simulink model "sus"  (Simulink 6.5)
settings: Solver=ode45  StartTime=0.0  StopTime=16  RelTol=1e-3
libraries: cdsFilt x266, cdsBitwise x92, cdsEpicsOut x84, cdsEpicsBinIn x56, cdsEpicsIn x20, cdsFiltCtrl x18, cdsMatrix x11, cdsSwitch x7, cdsWD x7, cdsFunctionCall x5, cdsRio1 x4, dac x3
(part 15 of 20)

== system sus/RLS/DELTA1 ==
  In1 : Inport
  time : Inport  Port=2
  delay_in : Inport  Port=3
  HOLD : Subsystem
  Sum2 : Sum  Inputs=+-
  dy1 : Outport
  delay_out : Outport  Port=2
  wires:
  HOLD/1(out) -> Sum2/2
  In1/1 -> Sum2/1, HOLD/1(In1)
  Sum2/1 -> dy1/1
  time/1 -> HOLD/2(time)
  HOLD/2(delay_out) -> delay_out/1
  delay_in/1 -> HOLD/3(delay_in)

== system sus/RLS/DELTA2 ==
  In1 : Inport
  time : Inport  Port=2
  delay_in : Inport  Port=3
  HOLD : Subsystem
  Sum2 : Sum  Inputs=+-
  dy1 : Outport
  delay_out : Outport  Port=2
  wires:
  HOLD/1(out) -> Sum2/2
  In1/1 -> Sum2/1, HOLD/1(In1)
  Sum2/1 -> dy1/1
  time/1 -> HOLD/2(time)
  HOLD/2(delay_out) -> delay_out/1
  delay_in/1 -> HOLD/3(delay_in)

== system sus/RLS/DELTA3 ==
  In1 : Inport
  time : Inport  Port=2
  delay_in : Inport  Port=3
  HOLD : Subsystem
  Sum2 : Sum  Inputs=+-
  dy1 : Outport
  delay_out : Outport  Port=2
  wires:
  HOLD/1(out) -> Sum2/2
  In1/1 -> Sum2/1, HOLD/1(In1)
  Sum2/1 -> dy1/1
  time/1 -> HOLD/2(time)
  HOLD/2(delay_out) -> delay_out/1
  delay_in/1 -> HOLD/3(delay_in)

== system sus/RLS/J11 ==
  In1 : Inport
  time : Inport  Port=2
  sattime : Inport  Port=3
  delay_in : Inport  Port=4
  Choice2 : Switch  Threshold=0.5
  HOLD : Subsystem
  SR : Constant  Value=0
  Sum2 : Sum
  out : Outport
  delay_out : Outport  Port=2
  wires:
  time/1 -> HOLD/2(time)
  HOLD/2(delay_out) -> delay_out/1
  delay_in/1 -> HOLD/3(delay_in)
  In1/1 -> Sum2/1
  Sum2/1 -> HOLD/1(In1)
  HOLD/1(out) -> Choice2/1
  sattime/1 -> Choice2/2
  Choice2/1 -> out/1, Sum2/2
  SR/1 -> Choice2/3

== system sus/RLS/J12 ==
  In1 : Inport
  time : Inport  Port=2
  sattime : Inport  Port=3
  delay_in : Inport  Port=4
  Choice2 : Switch  Threshold=0.5
  HOLD : Subsystem
  SR : Constant  Value=0
  Sum2 : Sum
  out : Outport
  delay_out : Outport  Port=2
  wires:
  time/1 -> HOLD/2(time)
  HOLD/2(delay_out) -> delay_out/1
  delay_in/1 -> HOLD/3(delay_in)
  In1/1 -> Sum2/1
  Sum2/1 -> HOLD/1(In1)
  HOLD/1(out) -> Choice2/1
  sattime/1 -> Choice2/2
  Choice2/1 -> out/1, Sum2/2
  SR/1 -> Choice2/3

== system sus/RLS/J21 ==
  In1 : Inport
  time : Inport  Port=2
  sattime : Inport  Port=3
  delay_in : Inport  Port=4
  Choice2 : Switch  Threshold=0.5
  HOLD : Subsystem
  SR : Constant  Value=0
  Sum2 : Sum
  out : Outport
  delay_out : Outport  Port=2
  wires:
  time/1 -> HOLD/2(time)
  HOLD/2(delay_out) -> delay_out/1
  delay_in/1 -> HOLD/3(delay_in)
  In1/1 -> Sum2/1
  Sum2/1 -> HOLD/1(In1)
  HOLD/1(out) -> Choice2/1
  sattime/1 -> Choice2/2
  Choice2/1 -> out/1, Sum2/2
  SR/1 -> Choice2/3

== system sus/RLS/J22 ==
  In1 : Inport
  time : Inport  Port=2
  sattime : Inport  Port=3
  delay_in : Inport  Port=4
  Choice2 : Switch  Threshold=0.5
  HOLD : Subsystem
  SR : Constant  Value=0
  Sum2 : Sum
  out : Outport
  delay_out : Outport  Port=2
  wires:
  time/1 -> HOLD/2(time)
  HOLD/2(delay_out) -> delay_out/1
  delay_in/1 -> HOLD/3(delay_in)
  In1/1 -> Sum2/1
  Sum2/1 -> HOLD/1(In1)
  HOLD/1(out) -> Choice2/1
  sattime/1 -> Choice2/2
  Choice2/1 -> out/1, Sum2/2
  SR/1 -> Choice2/3

== system sus/RLS/J31 ==
  In1 : Inport
  time : Inport  Port=2
  sattime : Inport  Port=3
  delay_in : Inport  Port=4
  Choice2 : Switch  Threshold=0.5
  HOLD : Subsystem
  SR : Constant  Value=0
  Sum2 : Sum
  out : Outport
  delay_out : Outport  Port=2
  wires:
  time/1 -> HOLD/2(time)
  HOLD/2(delay_out) -> delay_out/1
  delay_in/1 -> HOLD/3(delay_in)
  In1/1 -> Sum2/1
  Sum2/1 -> HOLD/1(In1)
  HOLD/1(out) -> Choice2/1
  sattime/1 -> Choice2/2
  Choice2/1 -> out/1, Sum2/2
  SR/1 -> Choice2/3

== system sus/RLS/J32 ==
  In1 : Inport
  time : Inport  Port=2
  sattime : Inport  Port=3
  delay_in : Inport  Port=4
  Choice2 : Switch  Threshold=0.5
  HOLD : Subsystem
  SR : Constant  Value=0
  Sum2 : Sum
  out : Outport
  delay_out : Outport  Port=2
  wires:
  time/1 -> HOLD/2(time)
  HOLD/2(delay_out) -> delay_out/1
  delay_in/1 -> HOLD/3(delay_in)
  In1/1 -> Sum2/1
  Sum2/1 -> HOLD/1(In1)
  HOLD/1(out) -> Choice2/1
  sattime/1 -> Choice2/2
  Choice2/1 -> out/1, Sum2/2
  SR/1 -> Choice2/3

== system sus/RLS/JHATDTHETA ==
  11 : Inport
  12 : Inport  Port=2
  21 : Inport  Port=3
  22 : Inport  Port=4
  31 : Inport  Port=5
  32 : Inport  Port=6
  dtheta1 : Inport  Port=7
  dtheta2 : Inport  Port=8
  Product{,1..5} (6 alike) : Product  RndMeth=Zero
  Sum : Sum  Inputs=|++
  Sum1 : Sum  Inputs=|++
  Sum2 : Sum  Inputs=|++
  dy1_hat : Outport
  dy2_hat : Outport  Port=2
  dy3_hat : Outport  Port=3
  wires:
  Product/1 -> Sum/1
  Sum/1 -> dy1_hat/1
  Product1/1 -> Sum/2
  Product2/1 -> Sum1/1
  Sum1/1 -> dy2_hat/1
  Product3/1 -> Sum1/2
  Product4/1 -> Sum2/1
  Sum2/1 -> dy3_hat/1
  Product5/1 -> Sum2/2
  dtheta1/1 -> Product/1, Product2/1, Product4/1
  dtheta2/1 -> Product1/1, Product3/1, Product5/1
  11/1 -> Product/2
  12/1 -> Product1/2
  21/1 -> Product2/2
  22/1 -> Product3/2
  31/1 -> Product4/2
  32/1 -> Product5/2

== system sus/RLS/K1 ==
  P11 : Inport
  P12 : Inport  Port=2
  P21 : Inport  Port=3
  P22 : Inport  Port=4
  dtheta1 : Inport  Port=5
  dtheta2 : Inport  Port=6
  lambda : Inport  Port=7
  Divide : Product  Inputs=*/  OutScaling=2^-10
  Divide1 : Product  Inputs=*/  OutScaling=2^-10
  PDTHETA : Subsystem
  Product : Product  RndMeth=Zero
  Product1 : Product  RndMeth=Zero
  Sum : Sum  Inputs=|+++
  K1_1 : Outport
  K1_2 : Outport  Port=2
  wires:
  P11/1 -> PDTHETA/1(P11)
  P12/1 -> PDTHETA/2(P12)
  P21/1 -> PDTHETA/3(P21)
  P22/1 -> PDTHETA/4(P22)
  dtheta1/1 -> PDTHETA/5(dtheta1), Product/2
  dtheta2/1 -> PDTHETA/6(dtheta2), Product1/2
  PDTHETA/1(out1) -> Product/1, Divide/1
  PDTHETA/2(out2) -> Product1/1, Divide1/1
  Product1/1 -> Sum/2
  Product/1 -> Sum/1
  lambda/1 -> Sum/3
  Sum/1 -> Divide/2, Divide1/2
  Divide/1 -> K1_1/1
  Divide1/1 -> K1_2/1

== system sus/RLS/K2 ==
  P11 : Inport
  P12 : Inport  Port=2
  P21 : Inport  Port=3
  P22 : Inport  Port=4
  dtheta1 : Inport  Port=5
  dtheta2 : Inport  Port=6
  lambda : Inport  Port=7
  Divide : Product  Inputs=*/  OutScaling=2^-10
  Divide1 : Product  Inputs=*/  OutScaling=2^-10
  PDTHETA : Subsystem
  Product : Product  RndMeth=Zero
  Product1 : Product  RndMeth=Zero
  Sum : Sum  Inputs=|+++
  K2_1 : Outport
  K2_2 : Outport  Port=2
  wires:
  P11/1 -> PDTHETA/1(P11)
  P12/1 -> PDTHETA/2(P12)
  P21/1 -> PDTHETA/3(P21)
  P22/1 -> PDTHETA/4(P22)
  dtheta1/1 -> PDTHETA/5(dtheta1), Product/2
  dtheta2/1 -> PDTHETA/6(dtheta2), Product1/2
  PDTHETA/1(out1) -> Product/1, Divide/1
  PDTHETA/2(out2) -> Product1/1, Divide1/1
  Product1/1 -> Sum/2
  Product/1 -> Sum/1
  lambda/1 -> Sum/3
  Sum/1 -> Divide/2, Divide1/2
  Divide/1 -> K2_1/1
  Divide1/1 -> K2_2/1

== system sus/RLS/K3 ==
  P11 : Inport
  P12 : Inport  Port=2
  P21 : Inport  Port=3
  P22 : Inport  Port=4
  dtheta1 : Inport  Port=5
  dtheta2 : Inport  Port=6
  lambda : Inport  Port=7
  Divide : Product  Inputs=*/  OutScaling=2^-10
  Divide1 : Product  Inputs=*/  OutScaling=2^-10
  PDTHETA : Subsystem
  Product : Product  RndMeth=Zero
  Product1 : Product  RndMeth=Zero
  Sum : Sum  Inputs=|+++
  K3_1 : Outport
  K3_2 : Outport  Port=2
  wires:
  P11/1 -> PDTHETA/1(P11)
  P12/1 -> PDTHETA/2(P12)
  P21/1 -> PDTHETA/3(P21)
  P22/1 -> PDTHETA/4(P22)
  dtheta1/1 -> PDTHETA/5(dtheta1), Product/2
  dtheta2/1 -> PDTHETA/6(dtheta2), Product1/2
  PDTHETA/1(out1) -> Product/1, Divide/1
  PDTHETA/2(out2) -> Product1/1, Divide1/1
  Product1/1 -> Sum/2
  Product/1 -> Sum/1
  lambda/1 -> Sum/3
  Sum/1 -> Divide/2, Divide1/2
  Divide/1 -> K3_1/1
  Divide1/1 -> K3_2/1

== system sus/RLS/P1 ==
  note: I - K*dtheta'
  note: (I - K*dtheta')*P
  K1_1 : Inport
  K1_2 : Inport  Port=2
  dtheta1 : Inport  Port=3
  dtheta2 : Inport  Port=4
  time : Inport  Port=5
  sattime : Inport  Port=6
  lambda : Inport  Port=7
  delay_In1 : Inport  Port=8
  delay_In2 : Inport  Port=9
  delay_In3 : Inport  Port=10
  delay_In4 : Inport  Port=11
  Choice{1..4} (4 alike) : Switch  Threshold=0.5
  Divide : Product  Inputs=*/  OutScaling=2^-10
  HOLD : Subsystem
  HOLD1 : Subsystem
  HOLD2 : Subsystem
  HOLD3 : Subsystem
  MATH : Subsystem
  MATH1 : Subsystem
  Product{1..4} (4 alike) : Product  RndMeth=Zero
  SR : Constant  Value=7
  SR1 : Constant  Value=0
  SR2 : Constant  Value=7
  SR3 : Constant  Value=0
  SR4 : Constant
  P1_11 : Outport
  P1_12 : Outport  Port=2
  P1_21 : Outport  Port=3
  P1_22 : Outport  Port=4
  delay_out1 : Outport  Port=5
  delay_out2 : Outport  Port=6
  delay_out3 : Outport  Port=7
  delay_out4 : Outport  Port=8
  wires:
  K1_1/1 -> MATH/1(K1_1)
  K1_2/1 -> MATH/2(K1_2)
  dtheta1/1 -> MATH/3(dtheta1)
  dtheta2/1 -> MATH/4(dtheta2)
  MATH/1(out11) -> MATH1/1(in11)
  MATH/2(out12) -> MATH1/2(in12)
  MATH/3(out21) -> MATH1/3(in21)
  MATH/4(out22) -> MATH1/4(in22)
  Choice2/1 -> HOLD/1(In1)
  sattime/1 -> Choice2/2, Choice1/2, Choice3/2, Choice4/2
  SR/1 -> Choice2/3
  MATH1/1(outP11) -> Choice2/1
  time/1 -> HOLD/2(time), HOLD2/2(time), HOLD3/2(time), HOLD1/2(time)
  Choice1/1 -> HOLD1/1(In1)
  SR1/1 -> Choice1/3
  MATH1/2(outP12) -> Choice1/1
  Choice4/1 -> HOLD2/1(In1)
  SR2/1 -> Choice4/3
  MATH1/3(outP21) -> Choice4/1
  Choice3/1 -> HOLD3/1(In1)
  SR3/1 -> Choice3/3
  MATH1/4(outP22) -> Choice3/1
  SR4/1 -> Divide/1
  lambda/1 -> Divide/2
  HOLD/1(out) -> Product2/2, P1_11/1
  HOLD1/1(out) -> Product1/2, P1_12/1
  HOLD2/1(out) -> Product3/2, P1_21/1
  HOLD3/1(out) -> Product4/2, P1_22/1
  Divide/1 -> Product2/1, Product1/1, Product4/1, Product3/1
  Product2/1 -> MATH1/5(P11)
  Product4/1 -> MATH1/8(P22)
  Product3/1 -> MATH1/7(P21)
  Product1/1 -> MATH1/6(P12)
  delay_In1/1 -> HOLD/3(delay_in)
  delay_In2/1 -> HOLD1/3(delay_in)
  delay_In3/1 -> HOLD2/3(delay_in)
  delay_In4/1 -> HOLD3/3(delay_in)
  HOLD/2(delay_out) -> delay_out1/1
  HOLD1/2(delay_out) -> delay_out2/1
  HOLD2/2(delay_out) -> delay_out3/1
  HOLD3/2(delay_out) -> delay_out4/1

== system sus/RLS/P2 ==
  note: I - K*dtheta'
  note: (I - K*dtheta')*P
  K1_1 : Inport
  K1_2 : Inport  Port=2
  dtheta1 : Inport  Port=3
  dtheta2 : Inport  Port=4
  time : Inport  Port=5
  sattime : Inport  Port=6
  lambda : Inport  Port=7
  delay_In1 : Inport  Port=8
  delay_In2 : Inport  Port=9
  delay_In3 : Inport  Port=10
  delay_In4 : Inport  Port=11
  Choice{1..4} (4 alike) : Switch  Threshold=0.5
  Divide : Product  Inputs=*/  OutScaling=2^-10
  HOLD : Subsystem
  HOLD1 : Subsystem
  HOLD2 : Subsystem
  HOLD3 : Subsystem
  MATH : Subsystem
  MATH1 : Subsystem
  Product{1..4} (4 alike) : Product  RndMeth=Zero
  SR : Constant  Value=7
  SR1 : Constant  Value=0
  SR2 : Constant  Value=7
  SR3 : Constant  Value=0
  SR4 : Constant
  P1_11 : Outport
  P1_12 : Outport  Port=2
  P1_21 : Outport  Port=3
  P1_22 : Outport  Port=4
  delay_out1 : Outport  Port=5
  delay_out2 : Outport  Port=6
  delay_out3 : Outport  Port=7
  delay_out4 : Outport  Port=8
  wires:
  K1_1/1 -> MATH/1(K1_1)
  K1_2/1 -> MATH/2(K1_2)
  dtheta1/1 -> MATH/3(dtheta1)
  dtheta2/1 -> MATH/4(dtheta2)
  MATH/1(out11) -> MATH1/1(in11)
  MATH/2(out12) -> MATH1/2(in12)
  MATH/3(out21) -> MATH1/3(in21)
  MATH/4(out22) -> MATH1/4(in22)
  Choice2/1 -> HOLD/1(In1)
  sattime/1 -> Choice2/2, Choice1/2, Choice3/2, Choice4/2
  SR/1 -> Choice2/3
  MATH1/1(outP11) -> Choice2/1
  time/1 -> HOLD/2(time), HOLD2/2(time), HOLD3/2(time), HOLD1/2(time)
  Choice1/1 -> HOLD1/1(In1)
  SR1/1 -> Choice1/3
  MATH1/2(outP12) -> Choice1/1
  Choice4/1 -> HOLD2/1(In1)
  SR2/1 -> Choice4/3
  MATH1/3(outP21) -> Choice4/1
  Choice3/1 -> HOLD3/1(In1)
  SR3/1 -> Choice3/3
  MATH1/4(outP22) -> Choice3/1
  SR4/1 -> Divide/1
  lambda/1 -> Divide/2
  HOLD/1(out) -> Product2/2, P1_11/1
  HOLD1/1(out) -> Product1/2, P1_12/1
  HOLD2/1(out) -> Product3/2, P1_21/1
  HOLD3/1(out) -> Product4/2, P1_22/1
  Divide/1 -> Product2/1, Product1/1, Product4/1, Product3/1
  Product2/1 -> MATH1/5(P11)
  Product4/1 -> MATH1/8(P22)
  Product3/1 -> MATH1/7(P21)
  Product1/1 -> MATH1/6(P12)
  delay_In1/1 -> HOLD/3(delay_in)
  delay_In2/1 -> HOLD1/3(delay_in)
  delay_In3/1 -> HOLD2/3(delay_in)
  delay_In4/1 -> HOLD3/3(delay_in)
  HOLD/2(delay_out) -> delay_out1/1
  HOLD1/2(delay_out) -> delay_out2/1
  HOLD2/2(delay_out) -> delay_out3/1
  HOLD3/2(delay_out) -> delay_out4/1

== system sus/RLS/P3 ==
  note: I - K*dtheta'
  note: (I - K*dtheta')*P
  K1_1 : Inport
  K1_2 : Inport  Port=2
  dtheta1 : Inport  Port=3
  dtheta2 : Inport  Port=4
  time : Inport  Port=5
  sattime : Inport  Port=6
  lambda : Inport  Port=7
  delay_In1 : Inport  Port=8
  delay_In2 : Inport  Port=9
  delay_In3 : Inport  Port=10
  delay_In4 : Inport  Port=11
  Choice{1..4} (4 alike) : Switch  Threshold=0.5
  Divide : Product  Inputs=*/  OutScaling=2^-10
  HOLD : Subsystem
  HOLD1 : Subsystem
  HOLD2 : Subsystem
  HOLD3 : Subsystem
  MATH : Subsystem
  MATH1 : Subsystem
  Product{1..4} (4 alike) : Product  RndMeth=Zero
  SR : Constant  Value=7
  SR1 : Constant  Value=0
  SR2 : Constant  Value=7
  SR3 : Constant  Value=0
  SR4 : Constant
  P1_11 : Outport
  P1_12 : Outport  Port=2
  P1_21 : Outport  Port=3
  P1_22 : Outport  Port=4
  delay_out1 : Outport  Port=5
  delay_out2 : Outport  Port=6
  delay_out3 : Outport  Port=7
  delay_out4 : Outport  Port=8
  wires:
  K1_1/1 -> MATH/1(K1_1)
  K1_2/1 -> MATH/2(K1_2)
  dtheta1/1 -> MATH/3(dtheta1)
  dtheta2/1 -> MATH/4(dtheta2)
  MATH/1(out11) -> MATH1/1(in11)
  MATH/2(out12) -> MATH1/2(in12)
  MATH/3(out21) -> MATH1/3(in21)
  MATH/4(out22) -> MATH1/4(in22)
  Choice2/1 -> HOLD/1(In1)
  sattime/1 -> Choice2/2, Choice1/2, Choice3/2, Choice4/2
  SR/1 -> Choice2/3
  MATH1/1(outP11) -> Choice2/1
  time/1 -> HOLD/2(time), HOLD2/2(time), HOLD3/2(time), HOLD1/2(time)
  Choice1/1 -> HOLD1/1(In1)
  SR1/1 -> Choice1/3
  MATH1/2(outP12) -> Choice1/1
  Choice4/1 -> HOLD2/1(In1)
  SR2/1 -> Choice4/3
  MATH1/3(outP21) -> Choice4/1
  Choice3/1 -> HOLD3/1(In1)
  SR3/1 -> Choice3/3
  MATH1/4(outP22) -> Choice3/1
  SR4/1 -> Divide/1
  lambda/1 -> Divide/2
  HOLD/1(out) -> Product2/2, P1_11/1
  HOLD1/1(out) -> Product1/2, P1_12/1
  HOLD2/1(out) -> Product3/2, P1_21/1
  HOLD3/1(out) -> Product4/2, P1_22/1
  Divide/1 -> Product2/1, Product1/1, Product4/1, Product3/1
  Product2/1 -> MATH1/5(P11)
  Product4/1 -> MATH1/8(P22)
  Product3/1 -> MATH1/7(P21)
  Product1/1 -> MATH1/6(P12)
  delay_In1/1 -> HOLD/3(delay_in)
  delay_In2/1 -> HOLD1/3(delay_in)
  delay_In3/1 -> HOLD2/3(delay_in)
  delay_In4/1 -> HOLD3/3(delay_in)
  HOLD/2(delay_out) -> delay_out1/1
  HOLD1/2(delay_out) -> delay_out2/1
  HOLD2/2(delay_out) -> delay_out3/1
  HOLD3/2(delay_out) -> delay_out4/1

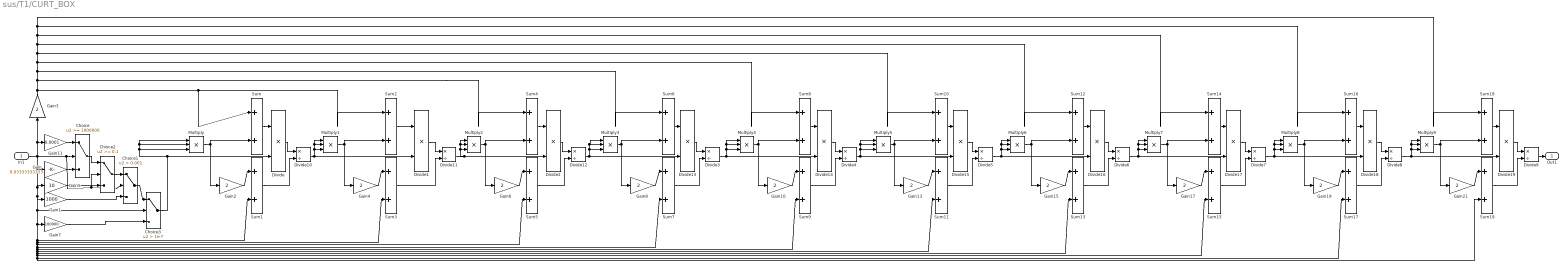
== system sus/T1/CURT_BOX ==
  In1 : Inport
  Choice : Switch  Threshold=1000000
  Choice1 : Switch  Criteria=u2 > Threshold  Threshold=0.001
  Choice2 : Switch  Threshold=0.1
  Choice3 : Switch  Criteria=u2 > Threshold  Threshold=1e-7
  Divide{,1..2,13..19} (10 alike) : Product  Inputs=**  OutScaling=2^-10
  Divide{3..12} (10 alike) : Product  Inputs=*/  OutScaling=2^-10
  Gain : Gain  Gain=0.03333333333
  Gain1 : Gain  Gain=1000
  Gain{2,4,6,8,10,13,15,17,19,21} (10 alike) : Gain  Gain=2
  Gain11 : Gain  Gain=0.0001
  Gain3 : Gain  Orientation=up  Gain=2
  Gain5 : Gain  Gain=10
  Gain7 : Gain  Gain=100000
  Multiply{,1..9} (10 alike) : Product  Inputs=***  OutScaling=2^-10
  Sum{,1..19} (20 alike) : Sum  Inputs=|++
  Out1 : Outport
  wires:
  In1/1 -> Gain/1, Gain1/1, Choice3/2, Sum1/2, Sum3/2, Sum5/2, Sum7/2, Sum9/2, Sum11/2, Sum13/2, Sum15/2, Sum17/2, Sum19/2, Gain7/1, Gain5/1, Choice/2, Choice2/2, Choice1/2, Gain11/1, Gain3/1
  Divide9/1 -> Out1/1
  Gain/1 -> Choice/3
  Gain11/1 -> Choice/1
  Choice3/1 -> Divide/2, Multiply/1, Multiply/2, Multiply/3
  Sum/1 -> Divide/1
  Multiply/1 -> Sum/2, Gain2/1
  Sum1/1 -> Divide10/2
  Gain2/1 -> Sum1/1
  Sum2/1 -> Divide1/1
  Multiply1/1 -> Sum2/2, Gain4/1
  Sum3/1 -> Divide11/2
  Gain4/1 -> Sum3/1
  Sum4/1 -> Divide2/1
  Multiply2/1 -> Sum4/2, Gain6/1
  Gain6/1 -> Sum5/1
  Divide12/1 -> Multiply3/1, Multiply3/2, Multiply3/3, Divide13/2
  Sum6/1 -> Divide13/1
  Multiply3/1 -> Sum6/2, Gain8/1
  Sum7/1 -> Divide3/2
  Gain8/1 -> Sum7/1
  Divide3/1 -> Multiply4/1, Multiply4/2, Multiply4/3, Divide14/2
  Sum8/1 -> Divide14/1
  Multiply4/1 -> Sum8/2, Gain10/1
  Sum9/1 -> Divide4/2
  Gain10/1 -> Sum9/1
  Divide4/1 -> Multiply5/1, Multiply5/2, Multiply5/3, Divide15/2
  Sum10/1 -> Divide15/1
  Multiply5/1 -> Sum10/2, Gain13/1
  Sum11/1 -> Divide5/2
  Gain13/1 -> Sum11/1
  Sum12/1 -> Divide16/1
  Multiply6/1 -> Sum12/2, Gain15/1
  Sum13/1 -> Divide6/2
  Gain15/1 -> Sum13/1
  Sum14/1 -> Divide17/1
  Multiply7/1 -> Sum14/2, Gain17/1
  Sum15/1 -> Divide7/2
  Gain17/1 -> Sum15/1
  Sum16/1 -> Divide18/1
  Multiply8/1 -> Sum16/2, Gain19/1
  Sum17/1 -> Divide8/2
  Gain19/1 -> Sum17/1
  Sum18/1 -> Divide19/1
  Multiply9/1 -> Sum18/2, Gain21/1
  Sum19/1 -> Divide9/2
  Gain21/1 -> Sum19/1
  Gain3/1 -> Sum16/1, Sum18/1, Sum14/1, Sum12/1, Sum10/1, Sum8/1, Sum6/1, Sum4/1, Sum2/1, Sum/1
  Divide/1 -> Divide10/1
  Divide10/1 -> Multiply1/1, Multiply1/2, Multiply1/3, Divide1/2
  Divide11/1 -> Divide2/2, Multiply2/1, Multiply2/2, Multiply2/3
  Divide1/1 -> Divide11/1
  Divide2/1 -> Divide12/1
  Sum5/1 -> Divide12/2
  Divide13/1 -> Divide3/1
  Divide14/1 -> Divide4/1
  Divide15/1 -> Divide5/1
  Divide5/1 -> Multiply6/1, Multiply6/2, Multiply6/3, Divide16/2
  Divide16/1 -> Divide6/1
  Divide6/1 -> Multiply7/1, Multiply7/2, Multiply7/3, Divide17/2
  Divide17/1 -> Divide7/1
  Divide7/1 -> Multiply8/1, Multiply8/2, Multiply8/3, Divide18/2
  Divide18/1 -> Divide8/1
  Divide8/1 -> Multiply9/1, Multiply9/2, Multiply9/3, Divide19/2
  Divide19/1 -> Divide9/1
  Gain1/1 -> Choice1/3
  Choice2/1 -> Choice1/1
  Choice/1 -> Choice2/1
  Gain5/1 -> Choice2/3
  Choice1/1 -> Choice3/1
  Gain7/1 -> Choice3/3

== system sus/T1/E2S ==
  In1 : Inport
  In2 : Inport  Port=2
  In3 : Inport  Port=3
  CONST1 : Constant
  CONST2 : Constant  Value=0
  CONST4 : Constant
  CONST5 : Constant  Value=0
  Choice1 : Switch  Criteria=u2 > Threshold  Threshold=0.0001
  Choice2 : Switch  Criteria=u2 > Threshold  Threshold=0.0001
  Choice3 : Switch  Criteria=u2 > Threshold
  Divide17 : Product  Inputs=*/  OutScaling=2^-10
  Product1 : Product  RndMeth=Zero
  Product35 : Product  RndMeth=Zero
  SQRT_BOX1 : Subsystem
  SQRT_BOX2 : Subsystem
  SQRT_BOX3 : Subsystem
  Out1 : Outport
  Out2 : Outport  Port=2
  Out3 : Outport  Port=3
  wires:
  SQRT_BOX1/1(Out1) -> Out1/1
  SQRT_BOX2/1(Out1) -> Out2/1
  SQRT_BOX3/1(Out1) -> Out3/1
  In1/1 -> Choice3/2, Choice3/1, SQRT_BOX1/1(In1)
  CONST4/1 -> Choice3/3
  Choice3/1 -> Divide17/2
  CONST1/1 -> Divide17/1
  In2/1 -> Product35/2, Choice1/1
  Divide17/1 -> Product35/1, Product1/1
  Product35/1 -> Choice1/2
  CONST5/1 -> Choice1/3
  Choice1/1 -> SQRT_BOX2/1(In1)
  In3/1 -> Choice2/1, Product1/2
  Product1/1 -> Choice2/2
  CONST2/1 -> Choice2/3
  Choice2/1 -> SQRT_BOX3/1(In1)

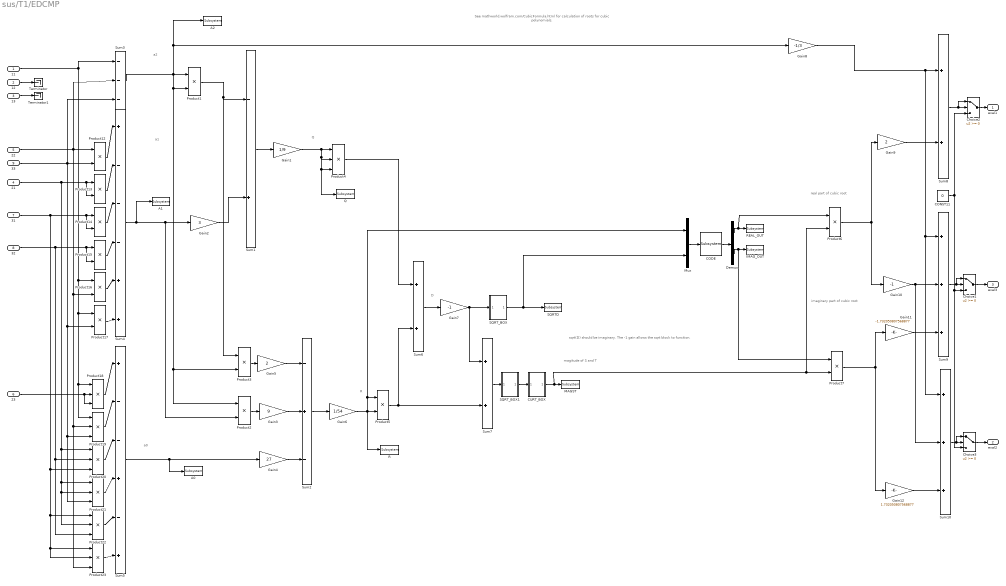
== system sus/T1/EDCMP ==
  note: a2
  note: a1
  note: a0
  note: Q
  note: R
  note: D
  note: sqrt(D) should be imaginary. The -1 gain allows the sqrt block to function.
  note: magitude of S and T
  note: real part of cubic root
  note: imaginary part of cubic root
  note: See mathworld.wolfram.com/CubicFormula.html for calculation of roots for cubic polynomials.
  11 : Inport
  12 : Inport  Port=2
  13 : Inport  Port=3
  21 : Inport  Port=4
  22 : Inport  Port=5
  23 : Inport  Port=6
  31 : Inport  Port=7
  32 : Inport  Port=8
  33 : Inport  Port=9
  A0 : cdsEpicsOut/Subsystem  Tag=cdsEpicsOutput  Description=|  SystemSampleTime=-1
      | Purpose:                                          
      | Output a FE signal to an EPICS channel.           
      |                                                   
      | Operation:                                        
      | Takes input value and passes it to EPICS record.  
      |                                                   
      | Usage:                                            
      | Name the part with the desired EPICS rrecord name.
      settings: AttributesFormatString=%<Tag>
  A1 : cdsEpicsOut/Subsystem  Tag=cdsEpicsOutput  Description=|  SystemSampleTime=-1
      | Purpose:                                          
      | Output a FE signal to an EPICS channel.           
      |                                                   
      | Operation:                                        
      | Takes input value and passes it to EPICS record.  
      |                                                   
      | Usage:                                            
      | Name the part with the desired EPICS rrecord name.
      settings: AttributesFormatString=%<Tag>
  A2 : cdsEpicsOut/Subsystem  Tag=cdsEpicsOutput  Description=|  SystemSampleTime=-1
      | Purpose:                                          
      | Output a FE signal to an EPICS channel.           
      |                                                   
      | Operation:                                        
      | Takes input value and passes it to EPICS record.  
      |                                                   
      | Usage:                                            
      | Name the part with the desired EPICS rrecord name.
      settings: AttributesFormatString=%<Tag>
  CODE : cdsFunctionCall/Subsystem  Tag=cdsFunctionCall  Description=|  SystemSampleTime=-1
      | Allows to make a call to external C function from the front-end code.                                            
      | User needs to use a Mux and a Demux to proved N number of inputs and M number of outputs to an external function.
      | Function "Foo()" code needs to be put in a file Foo.c in advLigo/src/fe/<model> directory.
      settings: AttributesFormatString=%<Tag>
  CONST11 : Constant  Value=0
  CURT_BOX : Subsystem
  Choice1 : Switch
  Choice2 : Switch
  Choice3 : Switch
  Demux : Demux  Outputs=2
  Gain1 : Gain  Gain=1/9
  Gain10 : Gain  Gain=-1
  Gain11 : Gain  Gain=-1.732050807568877
  Gain12 : Gain  Gain=1.732050807568877
  Gain2 : Gain  Gain=3
  Gain3 : Gain  Gain=9
  Gain4 : Gain  Gain=27
  Gain5 : Gain  Gain=2
  Gain6 : Gain  Gain=1/54
  Gain7 : Gain  Gain=-1
  Gain8 : Gain  Gain=-1/3
  Gain9 : Gain  Gain=2
  IMAG_OUT : cdsEpicsOut/Subsystem  Tag=cdsEpicsOutput  Description=|  SystemSampleTime=-1
      | Purpose:                                          
      | Output a FE signal to an EPICS channel.           
      |                                                   
      | Operation:                                        
      | Takes input value and passes it to EPICS record.  
      |                                                   
      | Usage:                                            
      | Name the part with the desired EPICS rrecord name.
      settings: AttributesFormatString=%<Tag>
  MAGST : cdsEpicsOut/Subsystem  Tag=cdsEpicsOutput  Description=|  SystemSampleTime=-1
      | Purpose:                                          
      | Output a FE signal to an EPICS channel.           
      |                                                   
      | Operation:                                        
      | Takes input value and passes it to EPICS record.  
      |                                                   
      | Usage:                                            
      | Name the part with the desired EPICS rrecord name.
      settings: AttributesFormatString=%<Tag>
  Mux : Mux  Inputs=2
  Product{1..3,5..7,12..17} (12 alike) : Product  RndMeth=Zero
  Product{4,18..23} (7 alike) : Product  Inputs=3  RndMeth=Zero
  Q : cdsEpicsOut/Subsystem  Tag=cdsEpicsOutput  Description=|  SystemSampleTime=-1
      | Purpose:                                          
      | Output a FE signal to an EPICS channel.           
      |                                                   
      | Operation:                                        
      | Takes input value and passes it to EPICS record.  
      |                                                   
      | Usage:                                            
      | Name the part with the desired EPICS rrecord name.
      settings: AttributesFormatString=%<Tag>
  R : cdsEpicsOut/Subsystem  Tag=cdsEpicsOutput  Description=|  SystemSampleTime=-1
      | Purpose:                                          
      | Output a FE signal to an EPICS channel.           
      |                                                   
      | Operation:                                        
      | Takes input value and passes it to EPICS record.  
      |                                                   
      | Usage:                                            
      | Name the part with the desired EPICS rrecord name.
      settings: AttributesFormatString=%<Tag>
  REAL_OUT : cdsEpicsOut/Subsystem  Tag=cdsEpicsOutput  Description=|  SystemSampleTime=-1
      | Purpose:                                          
      | Output a FE signal to an EPICS channel.           
      |                                                   
      | Operation:                                        
      | Takes input value and passes it to EPICS record.  
      |                                                   
      | Usage:                                            
      | Name the part with the desired EPICS rrecord name.
      settings: AttributesFormatString=%<Tag>
  SQRTD : cdsEpicsOut/Subsystem  Tag=cdsEpicsOutput  Description=|  SystemSampleTime=-1
      | Purpose:                                          
      | Output a FE signal to an EPICS channel.           
      |                                                   
      | Operation:                                        
      | Takes input value and passes it to EPICS record.  
      |                                                   
      | Usage:                                            
      | Name the part with the desired EPICS rrecord name.
      settings: AttributesFormatString=%<Tag>
  SQRT_BOX : Subsystem
  SQRT_BOX1 : Subsystem
  Sum1 : Sum  Inputs=-+
  Sum10 : Sum  Inputs=+++
  Sum2 : Sum  Inputs=-+-
  Sum3 : Sum  Inputs=|---
  Sum4 : Sum  Inputs=|+---++
  Sum5 : Sum  Inputs=|+--+-+
  Sum6 : Sum
  Sum7 : Sum
  Sum8 : Sum
  Sum9 : Sum  Inputs=+++
  Terminator : Terminator
  Terminator1 : Terminator
  eval1 : Outport
  eval2 : Outport  Port=2
  eval3 : Outport  Port=3
  wires:
  11/1 -> Sum3/1, Product16/1, Product17/1, Product18/1, Product19/1
  Product12/1 -> Sum4/1
  22/1 -> Product12/1, Product16/2, Product19/2, Product23/3, Sum3/2
  33/1 -> Product12/2, Product17/2, Product19/3, Product21/3, Sum3/3
  Product13/1 -> Sum4/2
  21/1 -> Product13/1, Product13/2, Product20/1, Product21/1, Product21/2, Product22/2
  Product14/1 -> Sum4/3
  31/1 -> Product14/1, Product14/2, Product20/3, Product22/1, Product23/1, Product23/2
  Product15/1 -> Sum4/4
  Product16/1 -> Sum4/5
  Product17/1 -> Sum4/6
  32/1 -> Product15/1, Product15/2, Product20/2, Product22/3
  Product18/1 -> Sum5/1
  23/1 -> Product18/2, Product18/3
  Product19/1 -> Sum5/2
  Product20/1 -> Sum5/3
  Product21/1 -> Sum5/4
  Product22/1 -> Sum5/5
  Product23/1 -> Sum5/6
  Sum4/1 -> Gain2/1, Product2/2, A1/1
  Sum3/1 -> Product1/1, Product1/2, Product2/1, Product3/2, Gain8/1, A2/1
  Product1/1 -> Sum1/1, Product3/1
  Gain2/1 -> Sum1/2
  Sum1/1 -> Gain1/1
  Product2/1 -> Gain3/1
  Sum5/1 -> Gain4/1, A0/1
  Gain4/1 -> Sum2/3
  Gain3/1 -> Sum2/2
  Gain5/1 -> Sum2/1
  Product3/1 -> Gain5/1
  Sum2/1 -> Gain6/1
  Gain1/1 -> Product4/1, Product4/2, Product4/3, Q/1
  Gain6/1 -> Product5/2, Product5/1, Mux/1, R/1
  Product4/1 -> Sum6/1
  Product5/1 -> Sum6/2, Sum7/2
  Sum6/1 -> Gain7/1
  Gain7/1 -> Sum7/1, SQRT_BOX/1(In1)
  Sum7/1 -> SQRT_BOX1/1(In1)
  SQRT_BOX1/1(Out1) -> CURT_BOX/1(In1)
  SQRT_BOX/1(Out1) -> SQRTD/1, Mux/2
  CURT_BOX/1(Out1) -> MAGST/1, Product6/2, Product7/2
  Demux/1 -> REAL_OUT/1, Product6/1
  Mux/1 -> CODE/1
  CODE/1 -> Demux/1
  Demux/2 -> IMAG_OUT/1, Product7/1
  Gain8/1 -> Sum8/1, Sum9/1, Sum10/1
  Gain9/1 -> Sum8/2
  Product6/1 -> Gain9/1, Gain10/1
  Gain10/1 -> Sum9/2, Sum10/2
  Gain11/1 -> Sum9/3
  Product7/1 -> Gain11/1, Gain12/1
  Gain12/1 -> Sum10/3
  12/1 -> Terminator/1
  13/1 -> Terminator1/1
  Choice2/1 -> eval1/1
  Sum8/1 -> Choice2/2, Choice2/1
  Sum9/1 -> Choice1/2, Choice1/1
  Sum10/1 -> Choice3/2, Choice3/1
  CONST11/1 -> Choice2/3, Choice1/3, Choice3/3
  Choice1/1 -> eval3/1
  Choice3/1 -> eval2/1
